simulink model "lscFP"  (Simulink 6.6)
settings: Solver=ode45  StartTime=0.0  StopTime=10.0  RelTol=1e-3
settings Model: Creator=Matt  LastModifiedBy=Matt

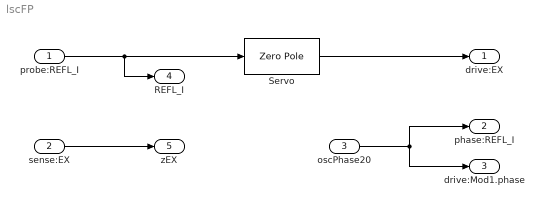
== system lscFP ==
  probe:REFL_I : Inport
  sense:EX : Inport  Port=2
  oscPhase20 : Inport  Port=3
  Servo : ZeroPole  Zeros=[-100]  Poles=[-1]  Gain=[1e-10]
  drive:EX : Outport
  phase:REFL_I : Outport  Port=2
  drive:Mod1.phase : Outport  Port=3
  REFL_I : Outport  Port=4
  zEX : Outport  Port=5
  wires:
  probe:REFL_I/1 -> Servo/1, REFL_I/1
  Servo/1 -> drive:EX/1
  sense:EX/1 -> zEX/1
  oscPhase20/1 -> phase:REFL_I/1, drive:Mod1.phase/1
